simulink model "tank"  (R2019b)
settings: Solver=ode45  StartTime=0.0  StopTime=inf  RelTol=1e-3  EnableMultiTasking=on
model workspace (MAT data in the model file):
  PLC_IP_Address = 'localhost'
libraries: sh_lib x74, nesl_utility x46, fl_lib x40, dspnetwork x33
(part 3 of 3)

== system tank/Virtual Gas Pipeline /The Gas Pipeline/Station 2 inlet valve ==
  valve : Inport
  Ball Valve : sh_lib/Valves/Flow Control Valves/Ball Valve  valve_seat_spec=1  cone_ang=120 deg  d_ball=18 in  d_orif=16 in  x_0=0 m  C_d=0.65  A_leak=1e-12 m^2  lam_spec=2  B_lam=0.999  Re_cr=10  flow_rate_specify=off  flow_rate_priority=None  flow_rate=0.001 m^3/s  flow_rate_nominal_specify=off  flow_rate_nominal_unit=m^3/s  flow_rate_nominal_value=1  pressure_drop_specify=off  pressure_drop_priority=None  pressure_drop=0 Pa  pressure_drop_nominal_specify=off  pressure_drop_nominal_unit=Pa  pressure_drop_nominal_value=1
      settings: SourceProductName=Simscape Fluids  SourceProductBaseCode=SH  InternalSimscapePortConfiguration="{\"Bottom\":[],\"Left\":[{\"id\":\"S\",\"label\":\"S\",\"type\":\"input\"},{\"id\":\"A\",\"label\":\"A\",\"type\":\"foundation.hydraulic.hydraulic\"}],\"Right\":[{\"id\":\"B\",\"label\":\"B\",\"type\":\"foundation.hydraulic.hydraulic\"}],\"Top\":[]}"
  Simulink-PS Converter : nesl_utility/Simulink-PS Converter  PhysicalDomain=network_engine_domain  SubClassName=ps_input  LeftPortType=input  RightPortType=output  PseudoPeriodic=off  Frequencies=[]  NoiseDistribution=none  NoiseParameters=[]  Unit=1  AffineConversion=off  FilteringAndDerivatives=zero  SimscapeFilterOrder=1  InputFilterTimeConstant=0.001  UdotUserProvided=1
  Inlet : PMIOPort  Side=Left
  outlet : PMIOPort  Port=2  Side=Right
  wires:
  valve/1 -> Simulink-PS Converter/1
  connections:
  Simulink-PS Converter/RConn1 -- Ball Valve/LConn1
  Inlet/RConn1 -- Ball Valve/LConn2
  outlet/RConn1 -- Ball Valve/RConn1

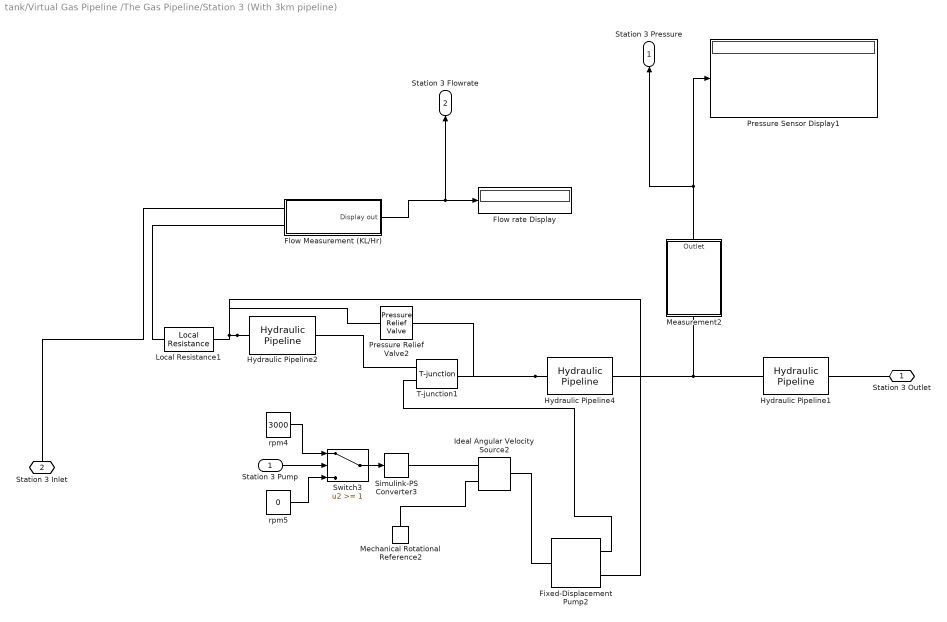
== system tank/Virtual Gas Pipeline /The Gas Pipeline/Station 3 (With 3km pipeline) ==
  Station 3 Pump : Inport
  Fixed-Displacement Pump2 : sh_lib/Pumps and Motors/Fixed-Displacement Pump  D=5e-4 m^3/rev  loss_spec=1  w_nominal=3000 rpm  pr_nominal=8.5 bar  visc_nominal=18 cSt  dens_nominal=900 kg/m^3  efficiency_vol=0.92  no_load_torque=0 N*m  torque_pressure_coeff=0.15915*(5e-4)*((0.92)/(0.8)-1 ) N*m/Pa  p_diff_eff_TLU=[100000, 1000000, 2000000] Pa  omega_eff_TLU=[25, 50, 100, 200, 300, 400] rad/s  vol_eff_TLU=[.816, .908, .954, .977, .981, .984; .325, .663, .831, .916, .925, .946; .137, .568, .78, .892, .893, .91]  mech_eff_TLU=[.996, .996, .996, .996, .996, .996; .988, .989, .989, .989, .989, .99; .981, .981, .982, .982, .983, .984]  p_diff_loss_TLU=[100000, 1000000, 2000000] Pa  omega_loss_TLU=[25, 50, 100, 200, 300, 400] rad/s  vol_loss_TLU=[.023, .023, .023, .023, .0285, .032; .0844, .0842, .0845, .084, .1125, .108; .1079, .108, .11, .108, .1605, .18] * 1e-3 m^3/s  mech_loss_TLU=[.002, .002, .002, .002, .002, .002; .0607, .0556, .0556, .0556, .0556, .0505; .1937, .1937, .1833, .1833, .1729, .1626] N*m  pressure_threshold=1e5 Pa  omega_threshold=10 rad/s  quadrant_check=0  pressure_check=0  min_valid_pressure=0 Pa  vol_eff_min=1e-3  vol_eff_max=1  mech_eff_min=1e-3  mech_eff_max=1
      settings: SourceProductName=Simscape Fluids  SourceProductBaseCode=SH  InternalSimscapePortConfiguration="{\"Bottom\":[],\"Left\":[{\"id\":\"S\",\"label\":\"S\",\"type\":\"foundation.mechanical.rotational.rotational\"}],\"Right\":[{\"id\":\"P\",\"label\":\"P\",\"type\":\"foundation.hydraulic.hydraulic\"},{\"id\":\"T\",\"label\":\"T\",\"type\":\"foundation.hydraulic.hydraulic\"}],\"Top\":[]}"
  Flow Measurement (KL/Hr) : Subsystem
  Flow rate Display : Display
  Hydraulic Pipeline1 : sh_lib/Pipelines/Hydraulic Pipeline  cs_type=1  d_in=16 in  area=1e-04 m^2  D_h=0.0112 m  s_factor=64  length=2900 m  length_ad=100 m  roughness=1.5e-3 m  Re_lam=2e+03  Re_turb=4e+03  wall_type=1  pr_r_coef=2e-12 m/Pa  time_const=0.01 s  k_sh=1.4  initial_pressure=0 Pa
      settings: SourceProductName=Simscape Fluids  SourceProductBaseCode=SH  InternalSimscapePortConfiguration="{\"Bottom\":[],\"Left\":[{\"id\":\"A\",\"label\":\"A\",\"type\":\"foundation.hydraulic.hydraulic\"}],\"Right\":[{\"id\":\"B\",\"label\":\"B\",\"type\":\"foundation.hydraulic.hydraulic\"}],\"Top\":[]}"
  Hydraulic Pipeline2 : sh_lib/Pipelines/Hydraulic Pipeline  cs_type=1  d_in=16 in  area=1e-04 m^2  D_h=0.0112 m  s_factor=64  length=500 m  length_ad=500 m  roughness=1.5e-3 m  Re_lam=2e+03  Re_turb=4e+03  wall_type=1  pr_r_coef=2e-12 m/Pa  time_const=0.01 s  k_sh=1.4  initial_pressure=0 Pa
      settings: SourceProductName=Simscape Fluids  SourceProductBaseCode=SH  InternalSimscapePortConfiguration="{\"Bottom\":[],\"Left\":[{\"id\":\"A\",\"label\":\"A\",\"type\":\"foundation.hydraulic.hydraulic\"}],\"Right\":[{\"id\":\"B\",\"label\":\"B\",\"type\":\"foundation.hydraulic.hydraulic\"}],\"Top\":[]}"
  Hydraulic Pipeline4 : sh_lib/Pipelines/Hydraulic Pipeline  cs_type=1  d_in=16 in  area=1e-04 m^2  D_h=0.0112 m  s_factor=64  length=100 m  length_ad=100 m  roughness=1.5e-3 m  Re_lam=2e+03  Re_turb=4e+03  wall_type=1  pr_r_coef=2e-12 m/Pa  time_const=0.01 s  k_sh=1.4  initial_pressure=0 Pa
      settings: SourceProductName=Simscape Fluids  SourceProductBaseCode=SH  InternalSimscapePortConfiguration="{\"Bottom\":[],\"Left\":[{\"id\":\"A\",\"label\":\"A\",\"type\":\"foundation.hydraulic.hydraulic\"}],\"Right\":[{\"id\":\"B\",\"label\":\"B\",\"type\":\"foundation.hydraulic.hydraulic\"}],\"Top\":[]}"
  Ideal Angular Velocity Source2 : fl_lib/Mechanical/Mechanical Sources/Ideal Angular Velocity Source
  Local Resistance1 : sh_lib/Local Hydraulic Resistances/Local Resistance  area=25.12 in^2  mdl_type=1  kp_d=2  kp_r=2  lam_spec=2  B_lam=0.999  Re_cr=150  Re_vec="[  -4e+03 -3e+03 -2e+03 -1000 -500 -200 -100 -50 -40 -30 -20 -15 -10 10 20 30 40 50 100 200 500 1000 2e+03 4e+03 5e+03 1e+04 ]"  loss_coeff_vec="[  0.25 0.3 0.65 0.9 0.65 0.75 0.9 1.15 1.35 1.65 2.3 2.8 3.1 5 2.7 1.8 1.46 1.3 0.9 0.65 0.42 0.3 0.2 0.4 0.42 0.25 ]"  interp_method=2  extrap_method=2  flow_rate_threshold=1e-6 m^3/s  flow_rate_specify=off  flow_rate_priority=None  flow_rate=0 m^3/s  flow_rate_nominal_specify=off  flow_rate_nominal_unit=m^3/s  flow_rate_nominal_value=1  pressure_drop_specify=off  pressure_drop_priority=None  pressure_drop=0 Pa  pressure_drop_nominal_specify=off  pressure_drop_nominal_unit=Pa  pressure_drop_nominal_value=1
      settings: SourceProductName=Simscape Fluids  SourceProductBaseCode=SH  InternalSimscapePortConfiguration="{\"Bottom\":[],\"Left\":[{\"id\":\"A\",\"label\":\"A\",\"type\":\"foundation.hydraulic.hydraulic\"}],\"Right\":[{\"id\":\"B\",\"label\":\"B\",\"type\":\"foundation.hydraulic.hydraulic\"}],\"Top\":[]}"
  Measurement2 : Subsystem
  Mechanical Rotational Reference2 : fl_lib/Mechanical/Rotational Elements/Mechanical Rotational Reference
  Pressure Relief Valve2 : sh_lib/Valves/Pressure Control Valves/Pressure Relief Valve  valve_area_spec=1  p_diff_TLU=[30.15e5 : 15e3 : 31.35e5] Pa  area_TLU=[1 : 1 : 9] .* 1e-5 m^2  area_max=157 in^2  pres_set=150 psi  reg_range=5 psi  C_d=0.7  A_leak=1e-12 m^2  lam_spec=2  B_lam=0.999  Re_cr=12  dynamic=0  tau=0.1 s  area_init=1e-12 m^2
      settings: SourceProductName=Simscape Fluids  SourceProductBaseCode=SH  InternalSimscapePortConfiguration="{\"Bottom\":[],\"Left\":[{\"id\":\"A\",\"label\":\"A\",\"type\":\"foundation.hydraulic.hydraulic\"}],\"Right\":[{\"id\":\"B\",\"label\":\"B\",\"type\":\"foundation.hydraulic.hydraulic\"}],\"Top\":[]}"
  Pressure Sensor Display1 : Display
  Simulink-PS Converter3 : nesl_utility/Simulink-PS Converter  PhysicalDomain=network_engine_domain  SubClassName=ps_input  LeftPortType=input  RightPortType=output  PseudoPeriodic=off  Frequencies=[]  NoiseDistribution=none  NoiseParameters=[]  Unit=1  AffineConversion=off  FilteringAndDerivatives=zero  SimscapeFilterOrder=1  InputFilterTimeConstant=0.001  UdotUserProvided=1
  Switch3 : Switch  Threshold=1
  T-junction1 : sh_lib/Local Hydraulic Resistances/T-junction  main_diam=16 in  branch_diam=16 in  kp_ab=1.12  kp_ba=1.12  kp_aa1=1.36  kp_a1a=1.65  kp_a1b=1.6  kp_ba1=1.8  lam_spec=2  B_lam=0.999  Re_cr=120
      settings: SourceProductName=Simscape Fluids  SourceProductBaseCode=SH  InternalSimscapePortConfiguration="{\"Bottom\":[],\"Left\":[{\"id\":\"A\",\"label\":\"A\",\"type\":\"foundation.hydraulic.hydraulic\"},{\"id\":\"A1\",\"label\":\"A1\",\"type\":\"foundation.hydraulic.hydraulic\"}],\"Right\":[{\"id\":\"B\",\"label\":\"B\",\"type\":\"foundation.hydraulic.hydraulic\"}],\"Top\":[]}"
  rpm4 : Constant  Value=3000
  rpm5 : Constant  Value=0
  Station 3 Outlet : PMIOPort  Side=Right
  Station 3 Inlet : PMIOPort  Port=2  Side=Left
  Station 3 Pressure : Outport
  Station 3 Flowrate : Outport  Port=2
  wires:
  rpm4/1 -> Switch3/1
  Switch3/1 -> Simulink-PS Converter3/1
  rpm5/1 -> Switch3/3
  Station 3 Pump/1 -> Switch3/2
  Measurement2/1(Outlet) -> Pressure Sensor Display1/1, Station 3 Pressure/1
  Flow Measurement (KL/Hr)/1(Display out) -> Flow rate Display/1, Station 3 Flowrate/1
  connections:
  T-junction1/LConn2 -- Fixed-Displacement Pump2/RConn1
  Mechanical Rotational Reference2/LConn1 -- Ideal Angular Velocity Source2/RConn2
  Ideal Angular Velocity Source2/LConn1 -- Fixed-Displacement Pump2/LConn1
  Simulink-PS Converter3/RConn1 -- Ideal Angular Velocity Source2/RConn1
  Measurement2/LConn1 -- Hydraulic Pipeline4/RConn1 -- Hydraulic Pipeline1/LConn1
  Hydraulic Pipeline2/RConn1 -- T-junction1/LConn1
  Hydraulic Pipeline2/LConn1 -- Local Resistance1/RConn1 -- Pressure Relief Valve2/RConn1 -- Fixed-Displacement Pump2/RConn2
  Hydraulic Pipeline4/LConn1 -- Pressure Relief Valve2/LConn1 -- T-junction1/RConn1
  Station 3 Inlet/RConn1 -- Flow Measurement (KL/Hr)/LConn1
  Hydraulic Pipeline1/RConn1 -- Station 3 Outlet/RConn1
  Flow Measurement (KL/Hr)/LConn2 -- Local Resistance1/LConn1

== system tank/Virtual Gas Pipeline /The Gas Pipeline/Station 3 inlet valve ==
  valve : Inport
  Ball Valve : sh_lib/Valves/Flow Control Valves/Ball Valve  valve_seat_spec=1  cone_ang=120 deg  d_ball=18 in  d_orif=16 in  x_0=0 m  C_d=0.65  A_leak=1e-12 m^2  lam_spec=2  B_lam=0.999  Re_cr=10  flow_rate_specify=off  flow_rate_priority=None  flow_rate=0.001 m^3/s  flow_rate_nominal_specify=off  flow_rate_nominal_unit=m^3/s  flow_rate_nominal_value=1  pressure_drop_specify=off  pressure_drop_priority=None  pressure_drop=0 Pa  pressure_drop_nominal_specify=off  pressure_drop_nominal_unit=Pa  pressure_drop_nominal_value=1
      settings: SourceProductName=Simscape Fluids  SourceProductBaseCode=SH  InternalSimscapePortConfiguration="{\"Bottom\":[],\"Left\":[{\"id\":\"S\",\"label\":\"S\",\"type\":\"input\"},{\"id\":\"A\",\"label\":\"A\",\"type\":\"foundation.hydraulic.hydraulic\"}],\"Right\":[{\"id\":\"B\",\"label\":\"B\",\"type\":\"foundation.hydraulic.hydraulic\"}],\"Top\":[]}"
  Simulink-PS Converter : nesl_utility/Simulink-PS Converter  PhysicalDomain=network_engine_domain  SubClassName=ps_input  LeftPortType=input  RightPortType=output  PseudoPeriodic=off  Frequencies=[]  NoiseDistribution=none  NoiseParameters=[]  Unit=1  AffineConversion=off  FilteringAndDerivatives=zero  SimscapeFilterOrder=1  InputFilterTimeConstant=0.001  UdotUserProvided=1
  Inlet : PMIOPort  Side=Left
  outlet : PMIOPort  Port=2  Side=Right
  wires:
  valve/1 -> Simulink-PS Converter/1
  connections:
  Simulink-PS Converter/RConn1 -- Ball Valve/LConn1
  Inlet/RConn1 -- Ball Valve/LConn2
  outlet/RConn1 -- Ball Valve/RConn1

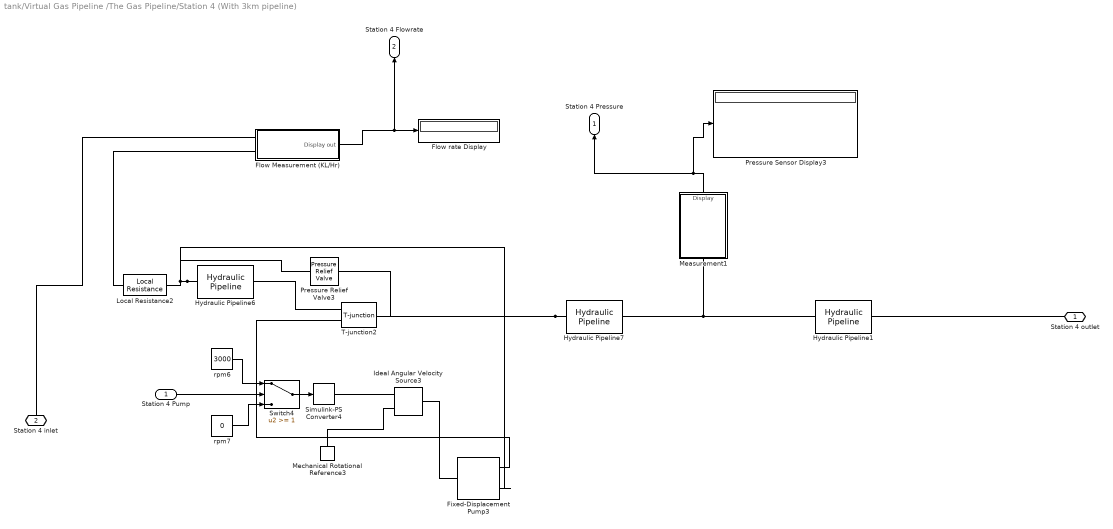
== system tank/Virtual Gas Pipeline /The Gas Pipeline/Station 4 (With 3km pipeline) ==
  "Station 4 Pump " : Inport
  Fixed-Displacement Pump3 : sh_lib/Pumps and Motors/Fixed-Displacement Pump  D=5e-4 m^3/rev  loss_spec=1  w_nominal=3000 rpm  pr_nominal=8.5 bar  visc_nominal=18 cSt  dens_nominal=900 kg/m^3  efficiency_vol=0.92  no_load_torque=0 N*m  torque_pressure_coeff=0.15915*(5e-4)*((0.92)/(0.8)-1 ) N*m/Pa  p_diff_eff_TLU=[100000, 1000000, 2000000] Pa  omega_eff_TLU=[25, 50, 100, 200, 300, 400] rad/s  vol_eff_TLU=[.816, .908, .954, .977, .981, .984; .325, .663, .831, .916, .925, .946; .137, .568, .78, .892, .893, .91]  mech_eff_TLU=[.996, .996, .996, .996, .996, .996; .988, .989, .989, .989, .989, .99; .981, .981, .982, .982, .983, .984]  p_diff_loss_TLU=[100000, 1000000, 2000000] Pa  omega_loss_TLU=[25, 50, 100, 200, 300, 400] rad/s  vol_loss_TLU=[.023, .023, .023, .023, .0285, .032; .0844, .0842, .0845, .084, .1125, .108; .1079, .108, .11, .108, .1605, .18] * 1e-3 m^3/s  mech_loss_TLU=[.002, .002, .002, .002, .002, .002; .0607, .0556, .0556, .0556, .0556, .0505; .1937, .1937, .1833, .1833, .1729, .1626] N*m  pressure_threshold=1e5 Pa  omega_threshold=10 rad/s  quadrant_check=0  pressure_check=0  min_valid_pressure=0 Pa  vol_eff_min=1e-3  vol_eff_max=1  mech_eff_min=1e-3  mech_eff_max=1
      settings: SourceProductName=Simscape Fluids  SourceProductBaseCode=SH  InternalSimscapePortConfiguration="{\"Bottom\":[],\"Left\":[{\"id\":\"S\",\"label\":\"S\",\"type\":\"foundation.mechanical.rotational.rotational\"}],\"Right\":[{\"id\":\"P\",\"label\":\"P\",\"type\":\"foundation.hydraulic.hydraulic\"},{\"id\":\"T\",\"label\":\"T\",\"type\":\"foundation.hydraulic.hydraulic\"}],\"Top\":[]}"
  Flow Measurement (KL/Hr) : Subsystem
  Flow rate Display : Display
  Hydraulic Pipeline1 : sh_lib/Pipelines/Hydraulic Pipeline  cs_type=1  d_in=16 in  area=1e-04 m^2  D_h=0.0112 m  s_factor=64  length=2900 m  length_ad=100 m  roughness=1.5e-3 m  Re_lam=2e+03  Re_turb=4e+03  wall_type=1  pr_r_coef=2e-12 m/Pa  time_const=0.01 s  k_sh=1.4  initial_pressure=0 Pa
      settings: SourceProductName=Simscape Fluids  SourceProductBaseCode=SH  InternalSimscapePortConfiguration="{\"Bottom\":[],\"Left\":[{\"id\":\"A\",\"label\":\"A\",\"type\":\"foundation.hydraulic.hydraulic\"}],\"Right\":[{\"id\":\"B\",\"label\":\"B\",\"type\":\"foundation.hydraulic.hydraulic\"}],\"Top\":[]}"
  Hydraulic Pipeline6 : sh_lib/Pipelines/Hydraulic Pipeline  cs_type=1  d_in=16 in  area=1e-04 m^2  D_h=0.0112 m  s_factor=64  length=500 m  length_ad=500 m  roughness=1.5e-3 m  Re_lam=2e+03  Re_turb=4e+03  wall_type=1  pr_r_coef=2e-12 m/Pa  time_const=0.01 s  k_sh=1.4  initial_pressure=0 Pa
      settings: SourceProductName=Simscape Fluids  SourceProductBaseCode=SH  InternalSimscapePortConfiguration="{\"Bottom\":[],\"Left\":[{\"id\":\"A\",\"label\":\"A\",\"type\":\"foundation.hydraulic.hydraulic\"}],\"Right\":[{\"id\":\"B\",\"label\":\"B\",\"type\":\"foundation.hydraulic.hydraulic\"}],\"Top\":[]}"
  Hydraulic Pipeline7 : sh_lib/Pipelines/Hydraulic Pipeline  cs_type=1  d_in=16 in  area=1e-04 m^2  D_h=0.0112 m  s_factor=64  length=100 m  length_ad=100 m  roughness=1.5e-3 m  Re_lam=2e+03  Re_turb=4e+03  wall_type=1  pr_r_coef=2e-12 m/Pa  time_const=0.01 s  k_sh=1.4  initial_pressure=0 Pa
      settings: SourceProductName=Simscape Fluids  SourceProductBaseCode=SH  InternalSimscapePortConfiguration="{\"Bottom\":[],\"Left\":[{\"id\":\"A\",\"label\":\"A\",\"type\":\"foundation.hydraulic.hydraulic\"}],\"Right\":[{\"id\":\"B\",\"label\":\"B\",\"type\":\"foundation.hydraulic.hydraulic\"}],\"Top\":[]}"
  Ideal Angular Velocity Source3 : fl_lib/Mechanical/Mechanical Sources/Ideal Angular Velocity Source
  Local Resistance2 : sh_lib/Local Hydraulic Resistances/Local Resistance  area=25.12 in^2  mdl_type=1  kp_d=2  kp_r=2  lam_spec=2  B_lam=0.999  Re_cr=150  Re_vec="[  -4e+03 -3e+03 -2e+03 -1000 -500 -200 -100 -50 -40 -30 -20 -15 -10 10 20 30 40 50 100 200 500 1000 2e+03 4e+03 5e+03 1e+04 ]"  loss_coeff_vec="[  0.25 0.3 0.65 0.9 0.65 0.75 0.9 1.15 1.35 1.65 2.3 2.8 3.1 5 2.7 1.8 1.46 1.3 0.9 0.65 0.42 0.3 0.2 0.4 0.42 0.25 ]"  interp_method=2  extrap_method=2  flow_rate_threshold=1e-6 m^3/s  flow_rate_specify=off  flow_rate_priority=None  flow_rate=0 m^3/s  flow_rate_nominal_specify=off  flow_rate_nominal_unit=m^3/s  flow_rate_nominal_value=1  pressure_drop_specify=off  pressure_drop_priority=None  pressure_drop=0 Pa  pressure_drop_nominal_specify=off  pressure_drop_nominal_unit=Pa  pressure_drop_nominal_value=1
      settings: SourceProductName=Simscape Fluids  SourceProductBaseCode=SH  InternalSimscapePortConfiguration="{\"Bottom\":[],\"Left\":[{\"id\":\"A\",\"label\":\"A\",\"type\":\"foundation.hydraulic.hydraulic\"}],\"Right\":[{\"id\":\"B\",\"label\":\"B\",\"type\":\"foundation.hydraulic.hydraulic\"}],\"Top\":[]}"
  Measurement1 : Subsystem
  Mechanical Rotational Reference3 : fl_lib/Mechanical/Rotational Elements/Mechanical Rotational Reference
  Pressure Relief Valve3 : sh_lib/Valves/Pressure Control Valves/Pressure Relief Valve  valve_area_spec=1  p_diff_TLU=[30.15e5 : 15e3 : 31.35e5] Pa  area_TLU=[1 : 1 : 9] .* 1e-5 m^2  area_max=157 in^2  pres_set=150 psi  reg_range=5 psi  C_d=0.7  A_leak=1e-12 m^2  lam_spec=2  B_lam=0.999  Re_cr=12  dynamic=0  tau=0.1 s  area_init=1e-12 m^2
      settings: SourceProductName=Simscape Fluids  SourceProductBaseCode=SH  InternalSimscapePortConfiguration="{\"Bottom\":[],\"Left\":[{\"id\":\"A\",\"label\":\"A\",\"type\":\"foundation.hydraulic.hydraulic\"}],\"Right\":[{\"id\":\"B\",\"label\":\"B\",\"type\":\"foundation.hydraulic.hydraulic\"}],\"Top\":[]}"
  Pressure Sensor Display3 : Display
  Simulink-PS Converter4 : nesl_utility/Simulink-PS Converter  PhysicalDomain=network_engine_domain  SubClassName=ps_input  LeftPortType=input  RightPortType=output  PseudoPeriodic=off  Frequencies=[]  NoiseDistribution=none  NoiseParameters=[]  Unit=1  AffineConversion=off  FilteringAndDerivatives=zero  SimscapeFilterOrder=1  InputFilterTimeConstant=0.001  UdotUserProvided=1
  Switch4 : Switch  Threshold=1
  T-junction2 : sh_lib/Local Hydraulic Resistances/T-junction  main_diam=16 in  branch_diam=16 in  kp_ab=1.12  kp_ba=1.12  kp_aa1=1.36  kp_a1a=1.65  kp_a1b=1.6  kp_ba1=1.8  lam_spec=2  B_lam=0.999  Re_cr=120
      settings: SourceProductName=Simscape Fluids  SourceProductBaseCode=SH  InternalSimscapePortConfiguration="{\"Bottom\":[],\"Left\":[{\"id\":\"A\",\"label\":\"A\",\"type\":\"foundation.hydraulic.hydraulic\"},{\"id\":\"A1\",\"label\":\"A1\",\"type\":\"foundation.hydraulic.hydraulic\"}],\"Right\":[{\"id\":\"B\",\"label\":\"B\",\"type\":\"foundation.hydraulic.hydraulic\"}],\"Top\":[]}"
  rpm6 : Constant  Value=3000
  rpm7 : Constant  Value=0
  Station 4 outlet : PMIOPort  Side=Right
  Station 4 inlet : PMIOPort  Port=2  Side=Left
  Station 4 Pressure : Outport
  Station 4 Flowrate : Outport  Port=2
  wires:
  Switch4/1 -> Simulink-PS Converter4/1
  rpm6/1 -> Switch4/1
  "Station 4 Pump "/1 -> Switch4/2
  rpm7/1 -> Switch4/3
  Measurement1/1(Display) -> Pressure Sensor Display3/1, Station 4 Pressure/1
  Flow Measurement (KL/Hr)/1(Display out) -> Station 4 Flowrate/1, Flow rate Display/1
  connections:
  T-junction2/LConn2 -- Fixed-Displacement Pump3/RConn1
  Mechanical Rotational Reference3/LConn1 -- Ideal Angular Velocity Source3/RConn2
  Simulink-PS Converter4/RConn1 -- Ideal Angular Velocity Source3/RConn1
  Hydraulic Pipeline6/LConn1 -- Local Resistance2/RConn1 -- Pressure Relief Valve3/RConn1 -- Fixed-Displacement Pump3/RConn2
  Hydraulic Pipeline7/LConn1 -- Pressure Relief Valve3/LConn1 -- T-junction2/RConn1
  Hydraulic Pipeline6/RConn1 -- T-junction2/LConn1
  Measurement1/LConn1 -- Hydraulic Pipeline7/RConn1 -- Hydraulic Pipeline1/LConn1
  Ideal Angular Velocity Source3/LConn1 -- Fixed-Displacement Pump3/LConn1
  Station 4 inlet/RConn1 -- Flow Measurement (KL/Hr)/LConn1
  Hydraulic Pipeline1/RConn1 -- Station 4 outlet/RConn1
  Flow Measurement (KL/Hr)/LConn2 -- Local Resistance2/LConn1

== system tank/Virtual Gas Pipeline /The Gas Pipeline/Station 4 inlet valve ==
  valve : Inport
  Ball Valve : sh_lib/Valves/Flow Control Valves/Ball Valve  valve_seat_spec=1  cone_ang=120 deg  d_ball=18 in  d_orif=16 in  x_0=0 m  C_d=0.65  A_leak=1e-12 m^2  lam_spec=2  B_lam=0.999  Re_cr=10  flow_rate_specify=off  flow_rate_priority=None  flow_rate=0.001 m^3/s  flow_rate_nominal_specify=off  flow_rate_nominal_unit=m^3/s  flow_rate_nominal_value=1  pressure_drop_specify=off  pressure_drop_priority=None  pressure_drop=0 Pa  pressure_drop_nominal_specify=off  pressure_drop_nominal_unit=Pa  pressure_drop_nominal_value=1
      settings: SourceProductName=Simscape Fluids  SourceProductBaseCode=SH  InternalSimscapePortConfiguration="{\"Bottom\":[],\"Left\":[{\"id\":\"S\",\"label\":\"S\",\"type\":\"input\"},{\"id\":\"A\",\"label\":\"A\",\"type\":\"foundation.hydraulic.hydraulic\"}],\"Right\":[{\"id\":\"B\",\"label\":\"B\",\"type\":\"foundation.hydraulic.hydraulic\"}],\"Top\":[]}"
  Simulink-PS Converter : nesl_utility/Simulink-PS Converter  PhysicalDomain=network_engine_domain  SubClassName=ps_input  LeftPortType=input  RightPortType=output  PseudoPeriodic=off  Frequencies=[]  NoiseDistribution=none  NoiseParameters=[]  Unit=1  AffineConversion=off  FilteringAndDerivatives=zero  SimscapeFilterOrder=1  InputFilterTimeConstant=0.001  UdotUserProvided=1
  Inlet : PMIOPort  Side=Left
  outlet : PMIOPort  Port=2  Side=Right
  wires:
  valve/1 -> Simulink-PS Converter/1
  connections:
  Simulink-PS Converter/RConn1 -- Ball Valve/LConn1
  Inlet/RConn1 -- Ball Valve/LConn2
  outlet/RConn1 -- Ball Valve/RConn1

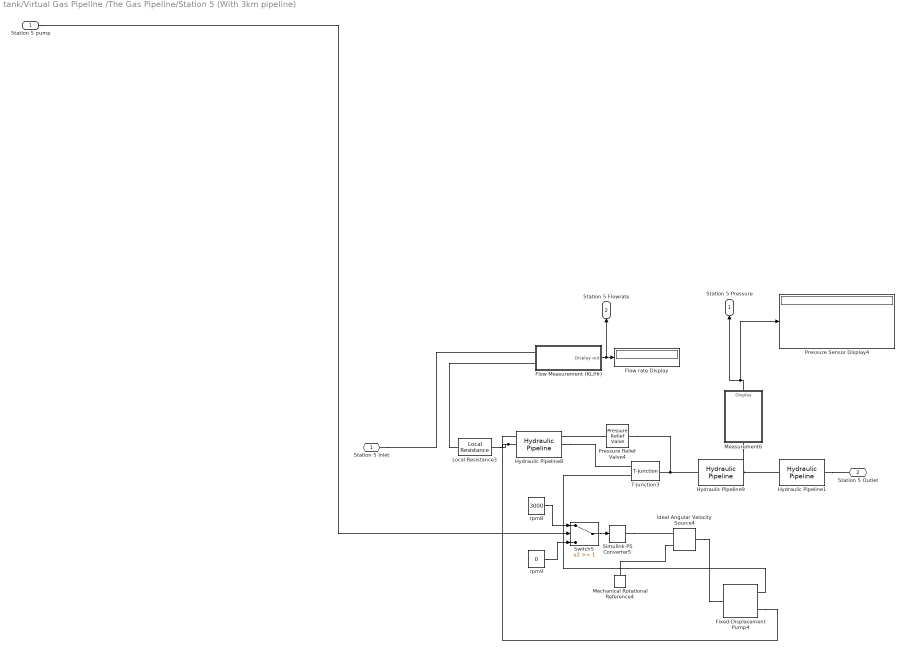
== system tank/Virtual Gas Pipeline /The Gas Pipeline/Station 5 (With 3km pipeline) ==
  Station 5 pump : Inport
  Fixed-Displacement Pump4 : sh_lib/Pumps and Motors/Fixed-Displacement Pump  D=5e-4 m^3/rev  loss_spec=1  w_nominal=3000 rpm  pr_nominal=8.5 bar  visc_nominal=18 cSt  dens_nominal=900 kg/m^3  efficiency_vol=0.92  no_load_torque=0 N*m  torque_pressure_coeff=0.15915*(5e-4)*((0.92)/(0.8)-1 ) N*m/Pa  p_diff_eff_TLU=[100000, 1000000, 2000000] Pa  omega_eff_TLU=[25, 50, 100, 200, 300, 400] rad/s  vol_eff_TLU=[.816, .908, .954, .977, .981, .984; .325, .663, .831, .916, .925, .946; .137, .568, .78, .892, .893, .91]  mech_eff_TLU=[.996, .996, .996, .996, .996, .996; .988, .989, .989, .989, .989, .99; .981, .981, .982, .982, .983, .984]  p_diff_loss_TLU=[100000, 1000000, 2000000] Pa  omega_loss_TLU=[25, 50, 100, 200, 300, 400] rad/s  vol_loss_TLU=[.023, .023, .023, .023, .0285, .032; .0844, .0842, .0845, .084, .1125, .108; .1079, .108, .11, .108, .1605, .18] * 1e-3 m^3/s  mech_loss_TLU=[.002, .002, .002, .002, .002, .002; .0607, .0556, .0556, .0556, .0556, .0505; .1937, .1937, .1833, .1833, .1729, .1626] N*m  pressure_threshold=1e5 Pa  omega_threshold=10 rad/s  quadrant_check=0  pressure_check=0  min_valid_pressure=0 Pa  vol_eff_min=1e-3  vol_eff_max=1  mech_eff_min=1e-3  mech_eff_max=1
      settings: SourceProductName=Simscape Fluids  SourceProductBaseCode=SH  InternalSimscapePortConfiguration="{\"Bottom\":[],\"Left\":[{\"id\":\"S\",\"label\":\"S\",\"type\":\"foundation.mechanical.rotational.rotational\"}],\"Right\":[{\"id\":\"P\",\"label\":\"P\",\"type\":\"foundation.hydraulic.hydraulic\"},{\"id\":\"T\",\"label\":\"T\",\"type\":\"foundation.hydraulic.hydraulic\"}],\"Top\":[]}"
  Flow Measurement (KL/Hr) : Subsystem
  Flow rate Display : Display
  Hydraulic Pipeline1 : sh_lib/Pipelines/Hydraulic Pipeline  cs_type=1  d_in=16 in  area=1e-04 m^2  D_h=0.0112 m  s_factor=64  length=2900 m  length_ad=100 m  roughness=1.5e-3 m  Re_lam=2e+03  Re_turb=4e+03  wall_type=1  pr_r_coef=2e-12 m/Pa  time_const=0.01 s  k_sh=1.4  initial_pressure=0 Pa
      settings: SourceProductName=Simscape Fluids  SourceProductBaseCode=SH  InternalSimscapePortConfiguration="{\"Bottom\":[],\"Left\":[{\"id\":\"A\",\"label\":\"A\",\"type\":\"foundation.hydraulic.hydraulic\"}],\"Right\":[{\"id\":\"B\",\"label\":\"B\",\"type\":\"foundation.hydraulic.hydraulic\"}],\"Top\":[]}"
  Hydraulic Pipeline8 : sh_lib/Pipelines/Hydraulic Pipeline  cs_type=1  d_in=16 in  area=1e-04 m^2  D_h=0.0112 m  s_factor=64  length=500 m  length_ad=500 m  roughness=1.5e-3 m  Re_lam=2e+03  Re_turb=4e+03  wall_type=1  pr_r_coef=2e-12 m/Pa  time_const=0.01 s  k_sh=1.4  initial_pressure=0 Pa
      settings: SourceProductName=Simscape Fluids  SourceProductBaseCode=SH  InternalSimscapePortConfiguration="{\"Bottom\":[],\"Left\":[{\"id\":\"A\",\"label\":\"A\",\"type\":\"foundation.hydraulic.hydraulic\"}],\"Right\":[{\"id\":\"B\",\"label\":\"B\",\"type\":\"foundation.hydraulic.hydraulic\"}],\"Top\":[]}"
  Hydraulic Pipeline9 : sh_lib/Pipelines/Hydraulic Pipeline  cs_type=1  d_in=16 in  area=1e-04 m^2  D_h=0.0112 m  s_factor=64  length=100 m  length_ad=100 m  roughness=1.5e-3 m  Re_lam=2e+03  Re_turb=4e+03  wall_type=1  pr_r_coef=2e-12 m/Pa  time_const=0.01 s  k_sh=1.4  initial_pressure=0 Pa
      settings: SourceProductName=Simscape Fluids  SourceProductBaseCode=SH  InternalSimscapePortConfiguration="{\"Bottom\":[],\"Left\":[{\"id\":\"A\",\"label\":\"A\",\"type\":\"foundation.hydraulic.hydraulic\"}],\"Right\":[{\"id\":\"B\",\"label\":\"B\",\"type\":\"foundation.hydraulic.hydraulic\"}],\"Top\":[]}"
  Ideal Angular Velocity Source4 : fl_lib/Mechanical/Mechanical Sources/Ideal Angular Velocity Source
  Local Resistance3 : sh_lib/Local Hydraulic Resistances/Local Resistance  area=25.12 in^2  mdl_type=1  kp_d=2  kp_r=2  lam_spec=2  B_lam=0.999  Re_cr=150  Re_vec="[  -4e+03 -3e+03 -2e+03 -1000 -500 -200 -100 -50 -40 -30 -20 -15 -10 10 20 30 40 50 100 200 500 1000 2e+03 4e+03 5e+03 1e+04 ]"  loss_coeff_vec="[  0.25 0.3 0.65 0.9 0.65 0.75 0.9 1.15 1.35 1.65 2.3 2.8 3.1 5 2.7 1.8 1.46 1.3 0.9 0.65 0.42 0.3 0.2 0.4 0.42 0.25 ]"  interp_method=2  extrap_method=2  flow_rate_threshold=1e-6 m^3/s  flow_rate_specify=off  flow_rate_priority=None  flow_rate=0 m^3/s  flow_rate_nominal_specify=off  flow_rate_nominal_unit=m^3/s  flow_rate_nominal_value=1  pressure_drop_specify=off  pressure_drop_priority=None  pressure_drop=0 Pa  pressure_drop_nominal_specify=off  pressure_drop_nominal_unit=Pa  pressure_drop_nominal_value=1
      settings: SourceProductName=Simscape Fluids  SourceProductBaseCode=SH  InternalSimscapePortConfiguration="{\"Bottom\":[],\"Left\":[{\"id\":\"A\",\"label\":\"A\",\"type\":\"foundation.hydraulic.hydraulic\"}],\"Right\":[{\"id\":\"B\",\"label\":\"B\",\"type\":\"foundation.hydraulic.hydraulic\"}],\"Top\":[]}"
  Measurement6 : Subsystem
  Mechanical Rotational Reference4 : fl_lib/Mechanical/Rotational Elements/Mechanical Rotational Reference
  Pressure Relief Valve4 : sh_lib/Valves/Pressure Control Valves/Pressure Relief Valve  valve_area_spec=1  p_diff_TLU=[30.15e5 : 15e3 : 31.35e5] Pa  area_TLU=[1 : 1 : 9] .* 1e-5 m^2  area_max=157 in^2  pres_set=150 psi  reg_range=5 psi  C_d=0.7  A_leak=1e-12 m^2  lam_spec=2  B_lam=0.999  Re_cr=12  dynamic=0  tau=0.1 s  area_init=1e-12 m^2
      settings: SourceProductName=Simscape Fluids  SourceProductBaseCode=SH  InternalSimscapePortConfiguration="{\"Bottom\":[],\"Left\":[{\"id\":\"A\",\"label\":\"A\",\"type\":\"foundation.hydraulic.hydraulic\"}],\"Right\":[{\"id\":\"B\",\"label\":\"B\",\"type\":\"foundation.hydraulic.hydraulic\"}],\"Top\":[]}"
  Pressure Sensor Display4 : Display
  Simulink-PS Converter5 : nesl_utility/Simulink-PS Converter  PhysicalDomain=network_engine_domain  SubClassName=ps_input  LeftPortType=input  RightPortType=output  PseudoPeriodic=off  Frequencies=[]  NoiseDistribution=none  NoiseParameters=[]  Unit=1  AffineConversion=off  FilteringAndDerivatives=zero  SimscapeFilterOrder=1  InputFilterTimeConstant=0.001  UdotUserProvided=1
  Switch5 : Switch  Threshold=1
  T-junction3 : sh_lib/Local Hydraulic Resistances/T-junction  main_diam=16 in  branch_diam=16 in  kp_ab=1.12  kp_ba=1.12  kp_aa1=1.36  kp_a1a=1.65  kp_a1b=1.6  kp_ba1=1.8  lam_spec=2  B_lam=0.999  Re_cr=120
      settings: SourceProductName=Simscape Fluids  SourceProductBaseCode=SH  InternalSimscapePortConfiguration="{\"Bottom\":[],\"Left\":[{\"id\":\"A\",\"label\":\"A\",\"type\":\"foundation.hydraulic.hydraulic\"},{\"id\":\"A1\",\"label\":\"A1\",\"type\":\"foundation.hydraulic.hydraulic\"}],\"Right\":[{\"id\":\"B\",\"label\":\"B\",\"type\":\"foundation.hydraulic.hydraulic\"}],\"Top\":[]}"
  rpm8 : Constant  Value=3000
  rpm9 : Constant  Value=0
  Station 5 Inlet : PMIOPort  Side=Left
  Station 5 Outlet : PMIOPort  Port=2  Side=Right
  Station 5 Pressure : Outport
  Station 5 Flowrate : Outport  Port=2
  wires:
  rpm9/1 -> Switch5/3
  Switch5/1 -> Simulink-PS Converter5/1
  rpm8/1 -> Switch5/1
  Station 5 pump/1 -> Switch5/2
  Measurement6/1(Display) -> Pressure Sensor Display4/1, Station 5 Pressure/1
  Flow Measurement (KL/Hr)/1(Display out) -> Station 5 Flowrate/1, Flow rate Display/1
  connections:
  Simulink-PS Converter5/RConn1 -- Ideal Angular Velocity Source4/RConn1
  T-junction3/LConn2 -- Fixed-Displacement Pump4/RConn1
  Hydraulic Pipeline8/RConn1 -- T-junction3/LConn1
  Hydraulic Pipeline8/LConn1 -- Local Resistance3/RConn1 -- Pressure Relief Valve4/RConn1 -- Fixed-Displacement Pump4/RConn2
  Mechanical Rotational Reference4/LConn1 -- Ideal Angular Velocity Source4/RConn2
  Ideal Angular Velocity Source4/LConn1 -- Fixed-Displacement Pump4/LConn1
  Station 5 Inlet/RConn1 -- Flow Measurement (KL/Hr)/LConn1
  Hydraulic Pipeline1/RConn1 -- Station 5 Outlet/RConn1
  Hydraulic Pipeline1/LConn1 -- Hydraulic Pipeline9/RConn1 -- Measurement6/LConn1
  Pressure Relief Valve4/LConn1 -- Hydraulic Pipeline9/LConn1 -- T-junction3/RConn1
  Flow Measurement (KL/Hr)/LConn2 -- Local Resistance3/LConn1

== system tank/Virtual Gas Pipeline /The Gas Pipeline/Station 5 inlet valve ==
  valve : Inport
  Ball Valve : sh_lib/Valves/Flow Control Valves/Ball Valve  valve_seat_spec=1  cone_ang=120 deg  d_ball=18 in  d_orif=16 in  x_0=0 m  C_d=0.65  A_leak=1e-12 m^2  lam_spec=2  B_lam=0.999  Re_cr=10  flow_rate_specify=off  flow_rate_priority=None  flow_rate=0.001 m^3/s  flow_rate_nominal_specify=off  flow_rate_nominal_unit=m^3/s  flow_rate_nominal_value=1  pressure_drop_specify=off  pressure_drop_priority=None  pressure_drop=0 Pa  pressure_drop_nominal_specify=off  pressure_drop_nominal_unit=Pa  pressure_drop_nominal_value=1
      settings: SourceProductName=Simscape Fluids  SourceProductBaseCode=SH  InternalSimscapePortConfiguration="{\"Bottom\":[],\"Left\":[{\"id\":\"S\",\"label\":\"S\",\"type\":\"input\"},{\"id\":\"A\",\"label\":\"A\",\"type\":\"foundation.hydraulic.hydraulic\"}],\"Right\":[{\"id\":\"B\",\"label\":\"B\",\"type\":\"foundation.hydraulic.hydraulic\"}],\"Top\":[]}"
  Simulink-PS Converter : nesl_utility/Simulink-PS Converter  PhysicalDomain=network_engine_domain  SubClassName=ps_input  LeftPortType=input  RightPortType=output  PseudoPeriodic=off  Frequencies=[]  NoiseDistribution=none  NoiseParameters=[]  Unit=1  AffineConversion=off  FilteringAndDerivatives=zero  SimscapeFilterOrder=1  InputFilterTimeConstant=0.001  UdotUserProvided=1
  Inlet : PMIOPort  Side=Left
  outlet : PMIOPort  Port=2  Side=Right
  wires:
  valve/1 -> Simulink-PS Converter/1
  connections:
  Simulink-PS Converter/RConn1 -- Ball Valve/LConn1
  Inlet/RConn1 -- Ball Valve/LConn2
  outlet/RConn1 -- Ball Valve/RConn1

== system tank/Virtual Gas Pipeline /The Gas Pipeline/Station 2 (With 3km pipeline)/Flow Measurement (KL//Hr) ==
  Constant : Constant  Value=3600
  Hydraulic Flow Rate Sensor : fl_lib/Hydraulic/Hydraulic Sensors/Hydraulic Flow Rate Sensor
      settings: SourceProductName=Simscape
  PS-Simulink Converter3 : nesl_utility/PS-Simulink Converter  PhysicalDomain=network_engine_domain  SubClassName=ps_output  LeftPortType=input  RightPortType=output  PseudoPeriodic=off  Frequencies=[]  Unit=m^3/s  AffineConversion=off
  Product : Product
  Inlet reference : PMIOPort  Side=Left
  " Outlet Reference" : PMIOPort  Port=2  Side=Left
  Display out : Outport
  wires:
  Product/1 -> Display out/1
  Constant/1 -> Product/2
  PS-Simulink Converter3/1 -> Product/1
  connections:
  PS-Simulink Converter3/LConn1 -- Hydraulic Flow Rate Sensor/RConn1
  Hydraulic Flow Rate Sensor/RConn2 -- " Outlet Reference"/RConn1
  Hydraulic Flow Rate Sensor/LConn1 -- Inlet reference/RConn1

== system tank/Virtual Gas Pipeline /The Gas Pipeline/Station 2 (With 3km pipeline)/Measurement3 ==
  Hydraulic Reference3 : fl_lib/Hydraulic/Hydraulic Elements/Hydraulic Reference
      settings: SourceProductName=Simscape
  Ideal Hydraulic Pressure Sensor3 : fl_lib/Hydraulic/Hydraulic Sensors/Hydraulic Pressure Sensor
      settings: SourceProductName=Simscape
  PS-Simulink Converter3 : nesl_utility/PS-Simulink Converter  PhysicalDomain=network_engine_domain  SubClassName=ps_output  LeftPortType=input  RightPortType=output  PseudoPeriodic=off  Frequencies=[]  Unit=Pa  AffineConversion=off
  Port : PMIOPort  Side=Left
  Display : Outport
  wires:
  PS-Simulink Converter3/1 -> Display/1
  connections:
  Ideal Hydraulic Pressure Sensor3/RConn1 -- Hydraulic Reference3/LConn1
  Ideal Hydraulic Pressure Sensor3/RConn2 -- PS-Simulink Converter3/LConn1
  Port/RConn1 -- Ideal Hydraulic Pressure Sensor3/LConn1

== system tank/Virtual Gas Pipeline /The Gas Pipeline/Station 3 (With 3km pipeline)/Flow Measurement (KL//Hr) ==
  Constant : Constant  Value=3600
  Hydraulic Flow Rate Sensor : fl_lib/Hydraulic/Hydraulic Sensors/Hydraulic Flow Rate Sensor
      settings: SourceProductName=Simscape
  PS-Simulink Converter3 : nesl_utility/PS-Simulink Converter  PhysicalDomain=network_engine_domain  SubClassName=ps_output  LeftPortType=input  RightPortType=output  PseudoPeriodic=off  Frequencies=[]  Unit=m^3/s  AffineConversion=off
  Product : Product
  Inlet reference : PMIOPort  Side=Left
  " Outlet Reference" : PMIOPort  Port=2  Side=Left
  Display out : Outport
  wires:
  Product/1 -> Display out/1
  Constant/1 -> Product/2
  PS-Simulink Converter3/1 -> Product/1
  connections:
  PS-Simulink Converter3/LConn1 -- Hydraulic Flow Rate Sensor/RConn1
  Hydraulic Flow Rate Sensor/RConn2 -- " Outlet Reference"/RConn1
  Hydraulic Flow Rate Sensor/LConn1 -- Inlet reference/RConn1

== system tank/Virtual Gas Pipeline /The Gas Pipeline/Station 3 (With 3km pipeline)/Measurement2 ==
  Hydraulic Reference3 : fl_lib/Hydraulic/Hydraulic Elements/Hydraulic Reference
      settings: SourceProductName=Simscape
  Ideal Hydraulic Pressure Sensor3 : fl_lib/Hydraulic/Hydraulic Sensors/Hydraulic Pressure Sensor
      settings: SourceProductName=Simscape
  PS-Simulink Converter3 : nesl_utility/PS-Simulink Converter  PhysicalDomain=network_engine_domain  SubClassName=ps_output  LeftPortType=input  RightPortType=output  PseudoPeriodic=off  Frequencies=[]  Unit=Pa  AffineConversion=off
  Inlet : PMIOPort  Side=Left
  Outlet : Outport
  wires:
  PS-Simulink Converter3/1 -> Outlet/1
  connections:
  Ideal Hydraulic Pressure Sensor3/RConn1 -- Hydraulic Reference3/LConn1
  Ideal Hydraulic Pressure Sensor3/RConn2 -- PS-Simulink Converter3/LConn1
  Inlet/RConn1 -- Ideal Hydraulic Pressure Sensor3/LConn1

== system tank/Virtual Gas Pipeline /The Gas Pipeline/Station 4 (With 3km pipeline)/Flow Measurement (KL//Hr) ==
  Constant : Constant  Value=3600
  Hydraulic Flow Rate Sensor : fl_lib/Hydraulic/Hydraulic Sensors/Hydraulic Flow Rate Sensor
      settings: SourceProductName=Simscape
  PS-Simulink Converter3 : nesl_utility/PS-Simulink Converter  PhysicalDomain=network_engine_domain  SubClassName=ps_output  LeftPortType=input  RightPortType=output  PseudoPeriodic=off  Frequencies=[]  Unit=m^3/s  AffineConversion=off
  Product : Product
  Inlet reference : PMIOPort  Side=Left
  " Outlet Reference" : PMIOPort  Port=2  Side=Left
  Display out : Outport
  wires:
  Product/1 -> Display out/1
  Constant/1 -> Product/2
  PS-Simulink Converter3/1 -> Product/1
  connections:
  PS-Simulink Converter3/LConn1 -- Hydraulic Flow Rate Sensor/RConn1
  Hydraulic Flow Rate Sensor/RConn2 -- " Outlet Reference"/RConn1
  Hydraulic Flow Rate Sensor/LConn1 -- Inlet reference/RConn1

== system tank/Virtual Gas Pipeline /The Gas Pipeline/Station 4 (With 3km pipeline)/Measurement1 ==
  Hydraulic Reference3 : fl_lib/Hydraulic/Hydraulic Elements/Hydraulic Reference
      settings: SourceProductName=Simscape
  Ideal Hydraulic Pressure Sensor3 : fl_lib/Hydraulic/Hydraulic Sensors/Hydraulic Pressure Sensor
      settings: SourceProductName=Simscape
  PS-Simulink Converter3 : nesl_utility/PS-Simulink Converter  PhysicalDomain=network_engine_domain  SubClassName=ps_output  LeftPortType=input  RightPortType=output  PseudoPeriodic=off  Frequencies=[]  Unit=Pa  AffineConversion=off
  Port : PMIOPort  Side=Left
  Display : Outport
  wires:
  PS-Simulink Converter3/1 -> Display/1
  connections:
  Ideal Hydraulic Pressure Sensor3/RConn1 -- Hydraulic Reference3/LConn1
  Ideal Hydraulic Pressure Sensor3/RConn2 -- PS-Simulink Converter3/LConn1
  Port/RConn1 -- Ideal Hydraulic Pressure Sensor3/LConn1

== system tank/Virtual Gas Pipeline /The Gas Pipeline/Station 5 (With 3km pipeline)/Flow Measurement (KL//Hr) ==
  Constant : Constant  Value=3600
  Hydraulic Flow Rate Sensor : fl_lib/Hydraulic/Hydraulic Sensors/Hydraulic Flow Rate Sensor
      settings: SourceProductName=Simscape
  PS-Simulink Converter3 : nesl_utility/PS-Simulink Converter  PhysicalDomain=network_engine_domain  SubClassName=ps_output  LeftPortType=input  RightPortType=output  PseudoPeriodic=off  Frequencies=[]  Unit=m^3/s  AffineConversion=off
  Product : Product
  Inlet reference : PMIOPort  Side=Left
  " Outlet Reference" : PMIOPort  Port=2  Side=Left
  Display out : Outport
  wires:
  Product/1 -> Display out/1
  Constant/1 -> Product/2
  PS-Simulink Converter3/1 -> Product/1
  connections:
  PS-Simulink Converter3/LConn1 -- Hydraulic Flow Rate Sensor/RConn1
  Hydraulic Flow Rate Sensor/RConn2 -- " Outlet Reference"/RConn1
  Hydraulic Flow Rate Sensor/LConn1 -- Inlet reference/RConn1

== system tank/Virtual Gas Pipeline /The Gas Pipeline/Station 5 (With 3km pipeline)/Measurement6 ==
  Hydraulic Reference3 : fl_lib/Hydraulic/Hydraulic Elements/Hydraulic Reference
      settings: SourceProductName=Simscape
  Ideal Hydraulic Pressure Sensor3 : fl_lib/Hydraulic/Hydraulic Sensors/Hydraulic Pressure Sensor
      settings: SourceProductName=Simscape
  PS-Simulink Converter3 : nesl_utility/PS-Simulink Converter  PhysicalDomain=network_engine_domain  SubClassName=ps_output  LeftPortType=input  RightPortType=output  PseudoPeriodic=off  Frequencies=[]  Unit=Pa  AffineConversion=off
  Port : PMIOPort  Side=Left
  Display : Outport
  wires:
  PS-Simulink Converter3/1 -> Display/1
  connections:
  Ideal Hydraulic Pressure Sensor3/RConn1 -- Hydraulic Reference3/LConn1
  Ideal Hydraulic Pressure Sensor3/RConn2 -- PS-Simulink Converter3/LConn1
  Port/RConn1 -- Ideal Hydraulic Pressure Sensor3/LConn1
